simulink model "MagLevTbx_UsbSerialPacketSend_Block"  (R2025b)
settings: Solver=FixedStepDiscrete  StartTime=0.0  StopTime=Inf  FixedStep=0.01  RelTol=1e-3  EnableMultiTasking=on
settings Model: ExtModeTrigDuration=2  Creator=riccardo  LastModifiedBy=riccardo
settings SolverCC: AutoInsertRateTranBlk=on
settings OptimizationCC: EnhancedBackFolding=on  PassReuseOutputArgsAs=Individual arguments  ZeroExternalMemoryAtStartup=off  ZeroInternalMemoryAtStartup=off  MaxStackSize=64  OptimizeBlockOrder=speed  DifferentSizesBufferReuse=on  OptimizationCustomize=off  EfficientTunableParamExpr=on
settings DebuggingCC: ParameterTunabilityLossMsg=error
settings HardwareCC: ProdBitPerPointer=32.0  ProdBitPerSizeT=32.0  ProdBitPerPtrDiffT=32.0  ProdLargestAtomicInteger=Long  ProdLargestAtomicFloat=Double  ProdWordSize=32.0  ProdHWDeviceType=ARM Compatible->ARM Cortex
settings SFSimCC: MATLABDynamicMemAlloc=off
settings RTWCC: SystemTargetFile=ert.tlc  HardwareBoard=Teensy 4.1 (Arduino Compatible)  TemplateMakefile=ert_default_tmf  Toolchain=Arduino ARM M7  BuildConfiguration=Faster Runs  Description=Embedded Coder
settings CodeAppCC: ForceParamTrailComments=on  IgnoreCustomStorageClasses=off  OperatorAnnotations=on  SimulinkDataObjDesc=on  SFDataObjDesc=on  InsertBlockDesc=on
settings ERTTargetCC: ExtModeTransport=3.0  ExtModeStaticAlloc=on  ExtModeAutomaticAllocSize=off  ExtModeStaticAllocSize=65536.0  ExtModeMexFile=ext_xcp  ExtModeIntrfLevel=Level2 - Open  InlinedParameterPlacement=Hierarchical  RootIOFormat=Structure reference  TargetLangStandard=C99 (ISO)  SupportContinuousTime=on  SupportVariableSizeSignals=on

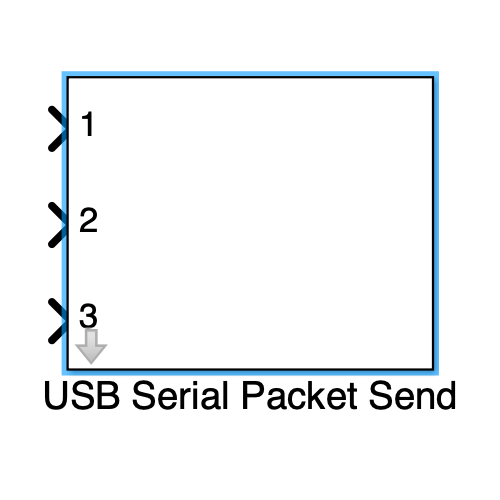
[thumbnail: Simulink's stored preview of the top-level diagram]
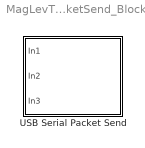
== system MagLevTbx_UsbSerialPacketSend_Block ==
  USB Serial Packet Send : Subsystem  mask(USB Serial Packet Send){waitDTR=on, packetSpec={'uint8', 'int16', 'single'}, cobsEncoded=on, nullTerminated=on, sampleTime=-1, showEnablePort=off}
      mask prompts: waitDTR "Wait for DTR signal"; packetSpec "Packet Specifier ( e.g. {'2*uint8', '3*single'} ):"; cobsEncoded "COBS Encoded"; nullTerminated "Null Terminated"; sampleTime "Sample time (-1 for inherited):"; showEnablePort "Show enable port"
      mask help: Send data packet using the USB serial port.
      mask init:
      | %   convert enable checkbox parameters to logical
      | cobsEncoded = logical(cobsEncoded);
      | nullTerminated = logical(nullTerminated);
      | waitDTR = logical(waitDTR);
      | 
      | %   init block
      | MagLevTbx_UsbSerialPacketSend_MaskInit(gcb, packetSpec, showEnablePort);
      mask Help:
      | Riccardo Antonello (riccardo.antonello@unipd.it)
      | 
      | February 18, 2026
      | 
      | Dept. of Information Engineering, University of Padova
      mask Callback sampleTime: MagLevTbx_UsbSerialPacketSend_MaskCbFcn_SampleTime();
      mask DialogControl Container4 Prompt: Communication link
      mask DialogControl Container3 Prompt: Packet definition

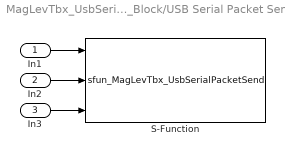
== system MagLevTbx_UsbSerialPacketSend_Block/USB Serial Packet Send ==
  In1 : Inport
  In2 : Inport  Port=2
  In3 : Inport  Port=3
  S-Function : S-Function  FunctionName=sfun_MagLevTbx_UsbSerialPacketSend  Parameters=packetSpec, cobsEncoded, nullTerminated, waitDTR, sampleTime  SFunctionDeploymentMode=off  EnableBusSupport=off
  wires:
  In1/1 -> S-Function/1
  In2/1 -> S-Function/2
  In3/1 -> S-Function/3
